simulink model "c28069_B2Bcontrol_hbF"  (R2018b)
settings: Solver=ode4  StartTime=0.0  StopTime=Inf  FixedStep=Ts/2  RelTol=1e-3
model workspace (MAT data in the model file):
  encoderResolution = 2000
  hallOffset = '0.5'
  indexOffset = 850
  polePairs = '4'
values from neighbouring files (symbols this model uses):
  g_adcA = 4.65/550    (= 0.00845454545455)    [data_init_B2B.m]
  g_adcB = 4.65/450    (= 0.0103333333333)    [data_init_B2B.m]
  imax = 10    [data_init_B2B.m]
  Ke = Kt    (= 0.0245)    [data_init_B2B.m]
  kiI = wcI*RaM    (= 3631.34782609)    [data_init_B2B.m]
  kiMR = kiI    (= 3631.34782609)    [data_init_B2B.m]
  kiW = wcW*B    (= 0.0131934782609)    [data_init_B2B.m]
  kpI = wcI*LaM    (= 5.78)    [data_init_B2B.m]
  kpMR = kpI    (= 5.78)    [data_init_B2B.m]
  kpW = wcW*J    (= 0.000749012608696)    [data_init_B2B.m]
  Kt = 0.0245    [data_init_B2B.m]
  LaM = 0.92e-3    (= 0.00092)    [data_init_B2B.m]
  maxBr = 0.05    [data_init_B2B.m]
  PWM_Counter_Period = CPU_frequency/PWM_frequency/2    (= 1500)    [data_init_B2B.m]
  PWM_CounterPeriod = PWM_Counter_Period    (= 1500)    [data_init_B2B.m]
  RaM = 0.578    [data_init_B2B.m]
  Ts = Tsw    (= 3.33333333333e-05)    [data_init_B2B.m]
  Tsm = Ts*5    (= 0.000166666666667)    [data_init_B2B.m]
  Tw = Ts*5    (= 0.000166666666667)    [data_init_B2B.m]
  Vdc = 10    [data_init_B2B.m]
  wmax = 250    [data_init_B2B.m]
undefined symbols (not defined in the file or in its folder): Down, GPTRIP1SEL, GPTRIP2SEL, Tss, TZ1, TZ2, Up
libraries: c2802xlib x9, simulink x9, peGeneralControl x4, c280xlib x3, c2806xlib x2
(part 2 of 2)

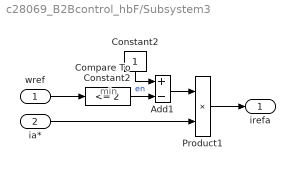
== system c28069_B2Bcontrol_hbF/Subsystem3 ==
  note: min
  wref : Inport
  ia* : Inport  Port=2
  Add1 : Sum  Inputs=+-
  Compare To Constant2 : simulink/Logic and Bit Operations/Compare To Constant  relop=<=  const=2  OutDataTypeStr=boolean
  Constant2 : Constant  OutDataTypeStr=single  SampleTime=Ts
  Product1 : Product
  irefa : Outport
  wires:
  ia*/1 -> Product1/2
  Constant2/1 -> Add1/1
  Add1/1 -> Product1/1
  Compare To Constant2/1 -> Add1/2  "en"
  Product1/1 -> irefa/1
  wref/1 -> Compare To Constant2/1

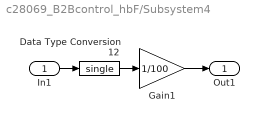
== system c28069_B2Bcontrol_hbF/Subsystem4 ==
  In1 : Inport
  Data Type Conversion12 : DataTypeConversion  OutDataTypeStr=single
  Gain1 : Gain  Gain=1/100
  Out1 : Outport
  wires:
  In1/1 -> Data Type Conversion12/1
  Gain1/1 -> Out1/1
  Data Type Conversion12/1 -> Gain1/1

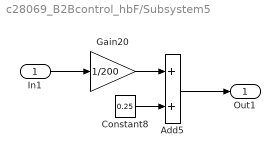
== system c28069_B2Bcontrol_hbF/Subsystem5 ==
  In1 : Inport
  Add5 : Sum
  Constant8 : Constant  Value=0.25  SampleTime=Ts
  Gain20 : Gain  Gain=1/200
  Out1 : Outport
  wires:
  Add5/1 -> Out1/1
  Gain20/1 -> Add5/1
  In1/1 -> Gain20/1
  Constant8/1 -> Add5/2

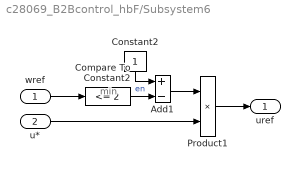
== system c28069_B2Bcontrol_hbF/Subsystem6 ==
  note: min
  wref : Inport
  u* : Inport  Port=2
  Add1 : Sum  Inputs=+-
  Compare To Constant2 : simulink/Logic and Bit Operations/Compare To Constant  relop=<=  const=2  OutDataTypeStr=boolean
  Constant2 : Constant  OutDataTypeStr=single  SampleTime=Ts
  Product1 : Product
  uref : Outport
  wires:
  wref/1 -> Compare To Constant2/1
  Product1/1 -> uref/1
  Compare To Constant2/1 -> Add1/2  "en"
  Add1/1 -> Product1/1
  Constant2/1 -> Add1/1
  u*/1 -> Product1/2

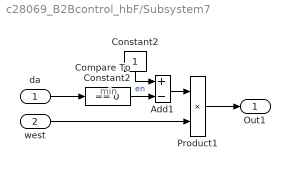
== system c28069_B2Bcontrol_hbF/Subsystem7 ==
  note: min
  da : Inport
  west : Inport  Port=2
  Add1 : Sum  Inputs=+-
  Compare To Constant2 : simulink/Logic and Bit Operations/Compare To Constant  relop===  const=0  OutDataTypeStr=boolean
  Constant2 : Constant  OutDataTypeStr=single
  Product1 : Product
  Out1 : Outport
  wires:
  west/1 -> Product1/2
  Constant2/1 -> Add1/1
  Add1/1 -> Product1/1
  Compare To Constant2/1 -> Add1/2  "en"
  Product1/1 -> Out1/1
  da/1 -> Compare To Constant2/1
